simulink model "ZOP_Main"  (R2018b)
settings: Solver=FixedStepDiscrete  StartTime=0.0  StopTime=inf  FixedStep=0.01  RelTol=1e-3
PostLoadFcn:
  | if any(exist('dsrtsu_mdlpostloadfcn', 'file') ~= 0), dsrtsu_mdlpostloadfcn('Execute', bdroot); end
values from neighbouring files (symbols this model uses):
  k_ZOP_ALC_Ramp = 1.0    [ZOP_Func.sldd]
  k_ZOP_LS_ChangingDist = 5.0    [ZOP_Func.sldd]
  k_ZOP_LS_ChangingTime = 0.5    [ZOP_Func.sldd]
  k_ZOP_SpdLmt_Enable = 1.0    [ZOP_Func.sldd]
  k_ZOP_V2X_Enable = 1.0    [ZOP_Func.sldd]
  k_ZOP_VcTJA_Enable = 1.0    [ZOP_Func.sldd]
  k_ZOP_VoiceAct_Enable = 1.0    [ZOP_Func.sldd]
  MODE_ZOP_ACTIVE = 3.0    [ZOP_Func.sldd]
  MODE_ZOP_FINISH = 10.0    [ZOP_Func.sldd]
  MODE_ZOP_LC = 7.0    [ZOP_Func.sldd]
(part 2 of 2)

== stateflow chart ZOP_Main/ZOP_Main_OS/ZOP_State_Machine ==
  state OFF
    en:
    ZOP_Mode = MODE_ZOP_OFF;
  state PASSIVE
    en:
    ZOP_Mode = MODE_ZOP_PASSIVE;
    ZOP_Vars = InitHoldState(ZOP_Vars);
    du:
    ZOP_Ready = CheckZopPreCondition(SystemCmd, VehStatus, MapInfo,...
    ACC_Status, LKS_Status);
  state FINISH
    en:
    ZOP_Mode = MODE_ZOP_FINISH;
    finishTimeCnt = 0;
    du:
    finishTimeCnt++;
  state ERROR
    en:
    ZOP_Mode = MODE_ZOP_ERROR;
    du:
    ;
  state READY
    en:
    ZOP_Mode = MODE_ZOP_READY;
    LaneChangeCmd = 0; ZOP_Finish = 0;
    LCRefDir = 0; LCDesDir = 0;
    du:
    ZOP_Ready = CheckZopPreCondition(SystemCmd, VehStatus, MapInfo,...
    ACC_Status, LKS_Status);
  state ENABLE
    en:
    ;
    du:
    ;
    state HOLD
      en:
      ZOP_Mode = MODE_ZOP_HOLD;
      LaneChangeCmd = 0; ZOP_Finish = 0;
      ZOP_Vars = InitHoldState(ZOP_Vars);
      % CheckLCResult();
      du:
      ZOP_Ready = CheckZopPreCondition(SystemCmd, VehStatus, MapInfo,...
      ACC_Status, LKS_Status);
      [LaneChangeCmd, LaneChangeDir, ZOP_Finish, ZOP_Vars] = CheckZopLCCondition(VehStatus, FusionObj,...
      FusionLane, MapInfo, RoadModel_Lane, RoadModel_TS, TgtObj, FObj, ZOP_Vars);
    state OVERIDE
      en:
      ZOP_Mode = MODE_ZOP_OVERIDE;
      du:
      ;
    state LANE_CHANGE
      en:
      ZOP_Mode = MODE_ZOP_LC;
      LaneChangeQuit = 0;
      ZOP_Vars = InitLCState(ZOP_Vars);
      du:
      [LaneChangeQuit, ZOP_Vars] = CheckZopLC(LaneChangeCmd, FusionObj,...
      FusionLane, MapInfo, RoadModel_Lane, LKS_Status, TgtObj, ZOP_Vars);
    (default) -> HOLD
    HOLD -> LANE_CHANGE [order 2] : [LaneChangeCmd == -1 || ...
        | LaneChangeCmd == 1]
    HOLD -> OVERIDE [order 1] : [ACC_Status.overide == 1 || ...
        | LKS_Status.overide == 1]
    LANE_CHANGE -> HOLD : [LaneChangeQuit]
    OVERIDE -> HOLD : [ACC_Status.overide == 0 && ...
        | LKS_Status.overide == 0]
  (default) -> OFF
  ERROR -> OFF [order 2] : [SystemCmd.SystemOn != 1]
  ENABLE -> OFF [order 4] : [SystemCmd.SystemOn != 1]
  READY -> OFF [order 1] : [SystemCmd.SystemOn != 1]
  FINISH -> OFF [order 1] : [SystemCmd.SystemOn != 1]
  OFF -> PASSIVE : [SystemCmd.SystemOn == 1]
  PASSIVE -> OFF [order 1] : [SystemCmd.SystemOn != 1]
  FINISH -> PASSIVE [order 2] : [finishTimeCnt >= 50]
  PASSIVE -> READY [order 2] : [ZOP_Ready == 1]
  READY -> PASSIVE [order 2] : [ZOP_Ready != 1]
  ENABLE -> FINISH [order 3] : [ZOP_Finish]
  ERROR -> READY [order 1] : [ACC_Status.error == 0 && ...
      | LKS_Status.error == 0]
  READY -> ERROR [order 3] : [ACC_Status.error == 1 || ...
      | LKS_Status.error == 1]
  READY -> ENABLE [order 4] : [ZOP_Ready == 1 ...
      | && SystemCmd.SystemEnable == 1 ...
      | && SystemCmd.SystemCancel != 1]
  ENABLE -> READY [order 2] : [ZOP_Ready != 1 ...
      | || SystemCmd.SystemCancel == 1]
  ENABLE -> ERROR [order 1] : [ACC_Status.error == 1 || ...
      | LKS_Status.error == 1]
  data: SystemCmd function_input Bus: SystemCmd_ST; VehStatus function_input Bus: VSI_VEHSTATE_ST; MapInfo function_input Bus: MapInfo_ST_Post; zop_ready function_output double; ACC_Status function_input Bus: ACC_Status_ST; LKS_Status function_input Bus: LKS_Status_ST; ZOPVars_in function_input Bus: ZOP_Var_ST; ZOPVars function_output Bus: ZOP_Var_ST; ZOPVars_in function_input Bus: ZOP_Var_ST; ZOPVars function_output Bus: ZOP_Var_ST; VehStatus function_input Bus: VSI_VEHSTATE_ST; FusionObj function_input Bus: FUS_OBJ_OUTPUT_ST; FusionLane function_input Bus: FUS_LANE_OUTPUT_ST; MapInfo function_input Bus: MapInfo_ST_Post; lc_cmd function_output int8; lc_pro function_output int8; ZOP_Finish function_output int8; RoadModel_Lane function_input Bus: LANEMODEL_OUTPUT_ST; RoadModel_TS function_input Bus: HWA_TARGETOBJECT_OUTPUT_ST; TgtObj function_input Bus: ZOP_Object_ST size=8; FObj function_input Bus: ZOP_Object_ST; ZOPVars_in function_input Bus: ZOP_Var_ST; ZOPVars function_output Bus: ZOP_Var_ST; k_ZOP_ALC_Enable parameter; k_ZOP_HoldCnt parameter; k_ZOP_LCProCnt parameter; k_ZOP_ALC_D10 parameter; k_ZOP_MapFlag_Enable parameter; k_ZOP_ALC_SCnt parameter; k_ZOP_ALC_SNCnt parameter; k_ZOP_ALC_SCnt_Thr parameter; k_ZOP_ALC_SpdEnable parameter; k_ZOP_SpdCkDstThr parameter; k_ZOP_ObjSpd_cf parameter; k_ZOP_SpdLoThr parameter; k_ZOP_SpdLoTimeThr parameter; k_ZOP_ALC_Ramp parameter; LCCmd function_input int8; FusionObj function_input Bus: FUS_OBJ_OUTPUT_ST; FusionLane function_input Bus: FUS_LANE_OUTPUT_ST; MapInfo function_input Bus: MapInfo_ST_Post; LC_Quit function_output int8; RoadModel_Lane function_input Bus: LANEMODEL_OUTPUT_ST; LKS_Status function_input Bus: LKS_Status_ST; TgtObj function_input Bus: ZOP_Object_ST size=8; ZOPVars_in function_input Bus: ZOP_Var_ST; ZOPVars function_output Bus: ZOP_Var_ST; k_ZOP_LCTimeMax parameter; k_ZOP_ALC_SCnt_LC parameter; k_ZOP_ALC_SNCnt_LC parameter; k_ZOP_ALC_SCnt_Thr_LC parameter; SystemCmd input Bus: SystemCmd_ST; VehStatus input Bus: VSI_VEHSTATE_ST; FusionObj input Bus: FUS_OBJ_OUTPUT_ST; FusionLane input Bus: FUS_LANE_OUTPUT_ST; RoadModel_Lane input Bus: LANEMODEL_OUTPUT_ST; RoadModel_TS input Bus: HWA_TARGETOBJECT_OUTPUT_ST; MapInfo input Bus: MapInfo_ST_Post; ACC_Status input Bus: ACC_Status_ST; LKS_Status input Bus: LKS_Status_ST; ZOP_Ready local int8; holdTimeCnt local int8; finishTimeCnt local int8; LaneChangeQuit local int8; LC_Succ local int8; LC_Fail local int8; lcTimeCnt local int8; ZOP_Mode output int8; ZOP_Finish output int8; LCPlanningState local int8; LaneChangeDcsn local int8; MODE_ZOP_ERROR parameter double; MODE_ZOP_FINISH parameter double; MODE_ZOP_HOLD parameter; MODE_ZOP_LC parameter; MODE_ZOP_OFF parameter; MODE_ZOP_OVERIDE parameter; MODE_ZOP_PASSIVE parameter; LCRefDir local int8; LCDesDir local int8; ZOP_Vars output Bus: ZOP_Var_ST; MODE_ZOP_READY parameter; TgtObj input Bus: ZOP_Object_ST size=8; LaneChangeCmd output int8; LaneChangeDir output int8; FObj input Bus: ZOP_Object_ST
  function zop_ready  = CheckZopPreCondition(SystemCmd, VehStatus, MapInfo,...:
    | function zop_ready  = CheckZopPreCondition(SystemCmd, VehStatus, MapInfo,...
    |     ACC_Status, LKS_Status)
    | 
    | zop_ready = 0;
    | if MapInfo.isInZopZone == 1 && (ACC_Status.ready || ACC_Status.active)...
    |         && (LKS_Status.ready || LKS_Status.active) % gear = D
    |     zop_ready = 1;
    | end
  function ZOPVars = InitHoldState(ZOPVars_in):
    | function ZOPVars = InitHoldState(ZOPVars_in)
    | 
    | ZOPVars = ZOPVars_in;
    | ZOPVars.LCRes = uint16(0);
    | ZOPVars.LCTip = uint16(0);
    | ZOPVars.LCNRes = uint16(0);
    | ZOPVars.DesLane = int8(0);
    | ZOPVars.LCDir = int8(0);
    | ZOPVars.holdTimeCnt = uint32(0);
    | ZOPVars.lcTimeCnt = uint32(0);
    | ZOPVars.lcProTimeCnt = uint32(0);
    | ZOPVars.lcDirCnt = uint32(0);
    | ZOPVars.Safe = int8(0);
    | ZOPVars.LSafeRaw = int8(0);
    | ZOPVars.LSafeCnt = int8(0);
    | ZOPVars.LSafeNCnt = int8(0);
    | ZOPVars.RSafeRaw = int8(0);
    | ZOPVars.RSafeCnt = int8(0);
    | ZOPVars.RSafeNCnt = int8(0);
    | ZOPVars.FinishState = int8(0);
    | ZOPVars.LCFailTip = int8(0);
    | ZOPVars.SpdTimeCnt(:) = uint32(0);
    | ZOPVars.SpdTmp(:) = single(100/3.6);
    | ZOPVars.Spd(:) = single(0/3.6);
    | ZOPVars.MapFlagDir = int8(0);
    | %ZOPVars.MapFlag = uint16(0);
  function ZOPVars = InitLCState(ZOPVars_in):
    | function ZOPVars = InitLCState(ZOPVars_in)
    | 
    | ZOPVars = ZOPVars_in;
    | ZOPVars.lcTimeCnt = uint32(0);
    | ZOPVars.Safe = int8(0);
    | ZOPVars.LSafeRaw = int8(0);
    | ZOPVars.LSafeCnt = int8(0);
    | ZOPVars.LSafeNCnt = int8(0);
    | ZOPVars.RSafeRaw = int8(0);
    | ZOPVars.RSafeCnt = int8(0);
    | ZOPVars.RSafeNCnt = int8(0);
    | ZOPVars.LCFailTip = int8(0);
  function [lc_cmd, lc_pro, ZOP_Finish, ZOPVars] = CheckZopLCCondition(VehStatus, FusionObj,...:
    | function [lc_cmd, lc_pro, ZOP_Finish, ZOPVars] = CheckZopLCCondition(VehStatus, FusionObj,...
    |     FusionLane, MapInfo, RoadModel_Lane, RoadModel_TS, TgtObj, FObj, ZOPVars_in)
    | 
    | ZOPVars = ZOPVars_in;
    | ZOPVars.LCRes = uint16(0);
    | ZOPVars.LCNRes = uint16(0);
    | ZOPVars.DesLane = int8(0);
    | ZOPVars.LCDir = int8(0);
    | ZOPVars.LCTime = single(8);
    | ZOPVars.LCCmd = int8(0);
    | lc_cmd = int8(0);
    | lc_pro = int8(0);
    | ZOP_Finish = int8(0);
    | ZOPVars.MapFlagDir = int8(0);
    | 
    | ZOPVars.LnHi = MapInfo.LaneNum;
    | ZOPVars.LnLo = int8(1);
    | if MapInfo.Dist2Dest > 3000
    |     ZOPVars.LnLo = min(MapInfo.LaneNum,min(2,MapInfo.LaneNum/2+1));
    |     %ZOPVars.DesLane = max(min(2,MapInfo.LaneNum), MapInfo.LaneIndex);
    | 	if MapInfo.Dist2Dest > 4000
    |         %ZOPVars.DesLane = max(int8(MapInfo.LaneNum/2+1),MapInfo.LaneIndex);
    |         ZOPVars.LnLo = min(MapInfo.LaneNum,int8(MapInfo.LaneNum/2+1));
    |     end
    | elseif MapInfo.Dist2Dest > 2500
    |     ZOPVars.LnHi = min(MapInfo.LaneNum,int8(MapInfo.LaneNum/2+1));
    |     %ZOPVars.DesLane = min(int8(MapInfo.LaneNum/2+1),MapInfo.LaneIndex);
    | else
    |     ZOPVars.LnHi = min(2,MapInfo.LaneNum);
    |     %ZOPVars.DesLane = min(2, MapInfo.LaneIndex);
    | 	if MapInfo.Dist2Dest < k_ZOP_ALC_D10
    |         ZOPVars.LnHi = int8(1);
    |         %ZOPVars.DesLane = int8(1);
    |     end
    | end
    | if MapInfo.Dist2Dest < 65534
    |     if MapInfo.LaneIndex < ZOPVars.LnLo
    |         ZOPVars.LCDir = int8(-1);
    |         ZOPVars.LCRes = uint16(4);
    |         ZOPVars.LCTip = uint16(5);
    |     elseif MapInfo.LaneIndex > ZOPVars.LnHi
    |         ZOPVars.LCDir = int8(1);
    |         ZOPVars.LCRes = uint16(2);
    |         ZOPVars.LCTip = uint16(3);
    |     end
    | end
    | 
    | % TODO:spd
    | ZOPVars.SpdTmp(:) = single(100/3.6);
    | if FObj.id > 0.5 && FObj.x < k_ZOP_SpdCkDstThr
    |     ZOPVars.SpdTmp(1) = FObj.vx+VehStatus.vRef;
    | end
    | for i=1:8
    |     if TgtObj(i).dir_f > 0 && TgtObj(i).dir < 0 && TgtObj(i).x < k_ZOP_SpdCkDstThr
    |         ZOPVars.SpdTmp(2) = min(ZOPVars.SpdTmp(2), TgtObj(i).vx+VehStatus.vRef);
    |     end
    |     if TgtObj(i).dir_f > 0 && TgtObj(i).dir > 0 && TgtObj(i).x < k_ZOP_SpdCkDstThr
    |         ZOPVars.SpdTmp(3) = min(ZOPVars.SpdTmp(3), TgtObj(i).vx+VehStatus.vRef);
    |     end
    | end
    | ZOPVars.Spd(1) = ZOPVars.SpdTmp(1)*k_ZOP_ObjSpd_cf + ZOPVars.Spd(1)*(1-k_ZOP_ObjSpd_cf);
    | ZOPVars.Spd(2) = ZOPVars.SpdTmp(2)*k_ZOP_ObjSpd_cf + ZOPVars.Spd(2)*(1-k_ZOP_ObjSpd_cf);
    | ZOPVars.Spd(3) = ZOPVars.SpdTmp(3)*k_ZOP_ObjSpd_cf + ZOPVars.Spd(3)*(1-k_ZOP_ObjSpd_cf);
    | if k_ZOP_ALC_SpdEnable > 0.5 && ZOPVars.LCDir == 0
    |     if ZOPVars.Spd(1) + k_ZOP_SpdLoThr < ZOPVars.Spd(2)
    |         ZOPVars.SpdTimeCnt(1) = ZOPVars.SpdTimeCnt(1) + uint32(1);
    |     else
    |         ZOPVars.SpdTimeCnt(1) = uint32(0);
    |     end
    |     if ZOPVars.Spd(1) + k_ZOP_SpdLoThr < ZOPVars.Spd(3)
    |         ZOPVars.SpdTimeCnt(2) = ZOPVars.SpdTimeCnt(2) + uint32(1);
    |     else
    |         ZOPVars.SpdTimeCnt(2) = uint32(0);
    |     end
    |     if ZOPVars.SpdTimeCnt(1) > k_ZOP_SpdLoTimeThr && MapInfo.LaneIndex+1 <= ZOPVars.LnHi
    |         ZOPVars.LCDir = int8(-1);
    |         ZOPVars.LCRes = uint16(1);
    |         ZOPVars.LCTip = uint16(1);
    |     % elseif ZOPVars.SpdTimeCnt(1) > k_ZOP_SpdLoTimeThr && MapInfo.LaneIndex+1 <= ZOPVars.LnHi
    |     end
    | end
    | 
    | % Ramp
    | if k_ZOP_ALC_Ramp > 0.5
    | %    if MapInfo.MapFlag ~= ZOPVars.MapFlag && (MapInfo.MapFlag == 1 || MapInfo.MapFlag == 2)
    |         if MapInfo.MapFlag == 1
    |             ZOPVars.MapFlagDir = int8(-1);
    |         elseif MapInfo.MapFlag == 2
    |             ZOPVars.MapFlagDir = int8(1);
    |         end
    | %    end
    |     if ZOPVars.MapFlagDir == -1 || ZOPVars.MapFlagDir == 1
    |         ZOPVars.LCDir = ZOPVars.MapFlagDir;
    | %         ZOPVars.LCCmd = ZOPVars.MapFlagDir;
    | %         lc_pro = ZOPVars.MapFlagDir;        
    |         ZOPVars.LCRes = uint16(2);
    |         ZOPVars.LCTip = uint16(3);
    | %         ZOPVars.lcProTimeCnt = ZOPVars.lcProTimeCnt + 1;
    | %         if ZOPVars.lcProTimeCnt > k_ZOP_LCProCnt/2
    | %             lc_cmd = ZOPVars.LCCmd;
    | %         end
    |     end
    |     ZOPVars.MapFlag = MapInfo.MapFlag;
    | else
    |     ZOPVars.MapFlag = uint16(0);
    | end
    | 
    | if k_ZOP_ALC_Ramp < 0.5 || ZOPVars.MapFlagDir == 0
    |     if MapInfo.LaneStable ~= 1
    |         ZOPVars.LCDir = int8(0);
    |         ZOPVars.LCNRes = ZOPVars.LCNRes + 1;
    |     end
    | end
    | if ZOPVars.LCDir == -1 && FusionLane.leftHostLane.type ~= 2 && ...
    |         FusionLane.leftHostLane.type ~= 6 && FusionLane.leftHostLane.type ~= 7
    |     ZOPVars.LCDir = int8(0);
    |     ZOPVars.LCNRes = ZOPVars.LCNRes + 2;
    | elseif ZOPVars.LCDir == 1 && FusionLane.rightHostLane.type ~= 2 && ...
    |         FusionLane.rightHostLane.type ~= 5 && FusionLane.rightHostLane.type ~= 7
    |     ZOPVars.LCDir = int8(0);
    |     ZOPVars.LCNRes = ZOPVars.LCNRes + 2;
    | end
    | 
    | ZOPVars.Safe = int8(0);
    | ZOPVars.LSafeRaw = int8(1);
    | ZOPVars.RSafeRaw = int8(1);
    | for i=1:8
    |     if TgtObj(i).dir == -1 && (TgtObj(i).exist(1) == 1 || TgtObj(i).exist(2) == 1)
    |         ZOPVars.LSafeRaw = int8(0);
    |     elseif TgtObj(i).dir == 1 && (TgtObj(i).exist(1) == 1 || TgtObj(i).exist(2) == 1)
    |         ZOPVars.RSafeRaw = int8(0);
    |     end
    | end
    | if ZOPVars.LSafeRaw == 1
    |     ZOPVars.LSafeCnt = min(ZOPVars.LSafeCnt+1, k_ZOP_ALC_SCnt);
    |     ZOPVars.LSafeNCnt = max(ZOPVars.LSafeNCnt-1, 0);
    | else
    |     ZOPVars.LSafeCnt = max(ZOPVars.LSafeCnt-1, 0);
    |     ZOPVars.LSafeNCnt = min(ZOPVars.LSafeNCnt+1, k_ZOP_ALC_SNCnt);
    | end
    | if ZOPVars.RSafeRaw == 1
    |     ZOPVars.RSafeCnt = min(ZOPVars.RSafeCnt+1, k_ZOP_ALC_SCnt);
    |     ZOPVars.RSafeNCnt = max(ZOPVars.RSafeNCnt-1, 0);
    | else
    |     ZOPVars.RSafeCnt = max(ZOPVars.RSafeCnt-1, 0);
    |     ZOPVars.RSafeNCnt = min(ZOPVars.RSafeNCnt+1, k_ZOP_ALC_SNCnt);
    | end
    | 
    | % if ZOPVars.SafeCnt > 20 && ZOPVars.SafeNCnt <= 5
    | %     ZOPVars.Safe = int8(1);
    | % elseif ZOPVars.SafeNCnt > 20 && ZOPVars.SafeCnt <= 5
    | %     ZOPVars.Safe = int8(-1);
    | % end
    | 
    | if ZOPVars.LCDir == -1
    |     if ZOPVars.LSafeCnt > k_ZOP_ALC_SCnt_Thr && ZOPVars.LSafeNCnt <= 3 && ZOPVars.LSafeRaw == 1
    |         %ZOPVars.Safe = int8(0);        
    |     else
    |         %ZOPVars.Safe = int8(-1);
    |         ZOPVars.LCDir = int8(0);
    |         ZOPVars.LCNRes = ZOPVars.LCNRes + 4;
    |     end
    | elseif ZOPVars.LCDir == 1
    |     if ZOPVars.RSafeCnt > k_ZOP_ALC_SCnt_Thr && ZOPVars.RSafeNCnt <= 3 && ZOPVars.RSafeRaw == 1
    |         %ZOPVars.Safe = int8(0);        
    |     else
    |         %ZOPVars.Safe = int8(-1);
    |         ZOPVars.LCDir = int8(0);
    |         ZOPVars.LCNRes = ZOPVars.LCNRes + 4;
    |     end
    | end
    | 
    | % if ZOPVars.Safe == 0
    | %     ZOPVars.LCDir = int8(0);
    | %     ZOPVars.LCNRes = ZOPVars.LCNRes + 4;
    | % end
    | % if ZOPVars.Safe == -1
    | %     ZOPVars.LCDir = int8(0);
    | %     ZOPVars.LCNRes = ZOPVars.LCNRes + 4;
    | % end
    | 
    | % time check
    | ZOP_HoldCnt = k_ZOP_HoldCnt;
    | if k_ZOP_ALC_Ramp > 0.5
    |     if MapInfo.MapFlag ~= 0
    |         ZOP_HoldCnt = single(10);
    |     else
    |         ZOP_HoldCnt = single(30);
    |     end
    | end
    | if ZOPVars.LCDir == 1 || ZOPVars.LCDir == -1
    |     if ZOPVars.holdTimeCnt > ZOP_HoldCnt
    |         ZOPVars.LCCmd = ZOPVars.LCDir;
    |         ZOPVars.lcDirCnt = ZOPVars.lcDirCnt+1;
    |     else
    |         ZOPVars.LCCmd = int8(0);
    |         ZOPVars.LCNRes = ZOPVars.LCNRes + 8;
    |     end
    | end
    | if MapInfo.MapFlag ~= 0 && k_ZOP_MapFlag_Enable > 0.5
    |     ZOPVars.LCCmd = int8(0);
    |     ZOPVars.LCNRes = ZOPVars.LCNRes + 256;
    | end
    | 
    | if ZOPVars.LCCmd == -1 || ZOPVars.LCCmd == 1
    |     lc_pro = ZOPVars.LCCmd;
    |     ZOPVars.lcProTimeCnt = ZOPVars.lcProTimeCnt + 1;
    | else
    |     ZOPVars.lcProTimeCnt = uint32(0);    
    |     ZOPVars.LCRes = uint16(0);
    |     ZOPVars.LCTip = uint16(0);
    | end
    | if (ZOPVars.lcProTimeCnt > k_ZOP_LCProCnt) || (k_ZOP_ALC_Ramp > 0.5 &&...
    |         ZOPVars.MapFlagDir ~= 0 && ZOPVars.lcProTimeCnt > k_ZOP_LCProCnt/3)
    |     lc_cmd = ZOPVars.LCCmd;
    | end
    | if k_ZOP_ALC_Enable < 0.5
    |     lc_cmd = int8(0);
    |     lc_pro = int8(0);
    |     ZOPVars.LCRes = uint16(0);
    |     ZOPVars.LCTip = uint16(0);
    | end
    | 
    | if k_ZOP_ALC_Ramp > 0.5
    |     if MapInfo.MapFlag == 128
    |         ZOPVars.FinishState = int8(1);
    |     end
    | else
    |     % Fail
    |     if (MapInfo.LocIndex == 1 || MapInfo.LocIndex == 3) && MapInfo.Dist2Dest < 400  && MapInfo.LaneIndex > 1
    |         ZOPVars.FinishState = int8(2);    % takeover
    |     elseif (MapInfo.LocIndex == 1 || MapInfo.LocIndex == 3) && MapInfo.Dist2Dest < 300  && MapInfo.LaneIndex == 1
    |         ZOPVars.FinishState = int8(1);
    |     end
    | end
    | ZOP_Finish = ZOPVars.FinishState;
    | ZOPVars.holdTimeCnt = ZOPVars.holdTimeCnt+1;
  function [LC_Quit, ZOPVars] = CheckZopLC(LCCmd, FusionObj,...:
    | function [LC_Quit, ZOPVars] = CheckZopLC(LCCmd, FusionObj,...
    |     FusionLane, MapInfo, RoadModel_Lane, LKS_Status, TgtObj, ZOPVars_in)
    | 
    | ZOPVars = ZOPVars_in;
    | ZOPVars.LCResult = int8(0);
    | 
    | ZOPVars.LSafeRaw = int8(1);
    | ZOPVars.RSafeRaw = int8(1);
    | for i=1:8
    |     if TgtObj(i).dir == -1 && (TgtObj(i).exist(1) == 1 || TgtObj(i).exist(2) == 1)
    |         ZOPVars.LSafeRaw = int8(0);
    |     elseif TgtObj(i).dir == 1 && (TgtObj(i).exist(1) == 1 || TgtObj(i).exist(2) == 1)
    |         ZOPVars.RSafeRaw = int8(0);
    |     end
    | end
    | if ZOPVars.LSafeRaw == 1
    |     ZOPVars.LSafeCnt = min(ZOPVars.LSafeCnt+1, k_ZOP_ALC_SCnt_LC);
    |     ZOPVars.LSafeNCnt = max(ZOPVars.LSafeNCnt-1, 0);
    | else
    |     ZOPVars.LSafeCnt = max(ZOPVars.LSafeCnt-1, 0);
    |     ZOPVars.LSafeNCnt = min(ZOPVars.LSafeNCnt+1, k_ZOP_ALC_SNCnt_LC);
    | end
    | if ZOPVars.RSafeRaw == 1
    |     ZOPVars.RSafeCnt = min(ZOPVars.RSafeCnt+1, k_ZOP_ALC_SCnt_LC);
    |     ZOPVars.RSafeNCnt = max(ZOPVars.RSafeNCnt-1, 0);
    | else
    |     ZOPVars.RSafeCnt = max(ZOPVars.RSafeCnt-1, 0);
    |     ZOPVars.RSafeNCnt = min(ZOPVars.RSafeNCnt+1, k_ZOP_ALC_SNCnt_LC);
    | end
    | 
    | if LKS_Status.lc_fail
    |     ZOPVars.LCResult = int8(-1);
    |     ZOPVars.LCFailTip = int8(4);
    | elseif LKS_Status.lc_finish
    |     ZOPVars.LCResult = int8(1);
    | elseif ZOPVars.lcTimeCnt*0.1 > k_ZOP_LCTimeMax
    |     ZOPVars.LCResult = int8(-1);
    | else
    |     if LCCmd == -1
    |         if ZOPVars.LSafeNCnt >= k_ZOP_ALC_SCnt_Thr_LC && ZOPVars.LSafeCnt <= 5 && ZOPVars.LSafeRaw == 0
    |             ZOPVars.LCResult = int8(-1);
    |             ZOPVars.LCFailTip = int8(1);
    |         end
    | %         for i=1:8
    | %             if TgtObj(i).dir == -1 && TgtObj(i).exist(2) == 1
    | %                 ZOPVars.LCResult = int8(-1);
    | %                 break;
    | %             end
    | %         end
    |     elseif LCCmd == 1
    |         if ZOPVars.RSafeNCnt >= k_ZOP_ALC_SCnt_Thr_LC && ZOPVars.RSafeCnt <= 5 && ZOPVars.RSafeRaw == 0
    |             ZOPVars.LCResult = int8(-1);
    |             ZOPVars.LCFailTip = int8(1);
    |         end
    | %         for i=1:8
    | %             if TgtObj(i).dir == 1 && TgtObj(i).exist(2) == 1
    | %                 ZOPVars.LCResult = int8(-1);
    | %                 break;
    | %             end
    | %         end
    |     end
    | end
    | 
    | ZOPVars.lcTimeCnt = ZOPVars.lcTimeCnt+1;
    | ZOPVars.LCDist = LKS_Status.lc_dist;
    | if ZOPVars.LCDist > 0 && ZOPVars.LCDist < 3.5
    |     ZOPVars.LCTime = 8*ZOPVars.LCDist/3.5;
    | else
    |     ZOPVars.LCTime = single(8);
    | end
    | 
    | if ZOPVars.LCResult ~= 0
    |     if ZOPVars.LCResult < 0
    |         ZOPVars.LCTip = uint16(7);
    |     end
    |     LC_Quit = int8(1);
    | else
    |     LC_Quit = int8(0);
    | end

== stateflow chart ZOP_Main/ZOP_OS ==
  settings: sampleTime=0.005
  (default) -> (junction 1) : {
      | i = i+1;
      | }
  (junction 1) -> (junction 22) [order 1] : [i %% 2 == 0]
  (junction 22) -> (junction 4) : {
      | do_ZOP_CAN;
      | do_LightLogic;
      | }
  (junction 1) -> (junction 4) [order 2]
  (junction 4) -> (junction 7) [order 1] : [i >= 10]
  (junction 4) -> (junction 6) [order 2]
  (junction 7) -> (junction 8) : {
      | do_LKS_CONV;
      | do_ZOP_Feature;
      | i = 0;
      | }
  (junction 8) -> (junction 6)
  (junction 6) -> (junction 13)
  data: i local int32
  events: do_ZOP_CAN output FUNCTION_CALL_EVENT; do_LightLogic output FUNCTION_CALL_EVENT; do_ZOP_Feature output FUNCTION_CALL_EVENT; do_LKS_CONV output FUNCTION_CALL_EVENT

== stateflow chart ZOP_Main/ZOP_Main_OS/LaneStateProcess ==
  settings: description=_0p0.DUMMY.222_000_
  state STABLE
    en:
    LaneStable = (LaneCur != 0);
    LaneCurPost = LaneCur;
    du:
    LaneStable = (LaneCur != 0);
  state CHANGING
    en:
    LaneStable = 0;
    changingCnt = 0;
    du:
    changingCnt++;
  state INIT
    en:
    LaneStable = 0;
    LaneCurPost = LaneCur;
  STABLE -> INIT [order 1] : [!ZOP_Enable]
  STABLE -> CHANGING [order 2] : [LaneNum_last != LaneNum ...
      | || LaneCur_last != LaneCur ...
      | || LCState == MODE_ZOP_LC]
  CHANGING -> STABLE [order 2] : [changingCnt*0.1 > k_LS_ChangingTime ...
      | && VehSpeed_mps*changingCnt*0.1 > k_LS_ChangingDist]
  CHANGING -> CHANGING [order 1] : [LaneCur_last != LaneCur ...
      | || LaneNum_last != LaneNum ...
      | || LCState == MODE_ZOP_LC]
  INIT -> CHANGING : [ZOP_Enable]
  CHANGING -> INIT [order 3] : [!ZOP_Enable]
  (default) -> INIT
  data: ZOP_Enable input; LaneCurPost output; changingCnt local int32; LaneCur input; LaneCur_last input; LCState input; VehSpeed_mps input; LaneStable output; LaneNum input; LaneNum_last input; k_LS_ChangingDist input; k_LS_ChangingTime input; MODE_ZOP_LC parameter

== stateflow chart ZOP_Main/ZOP_Main_OS/TargetCheck ==
  state DEFAULT
    en:
    ;
    du:
    [ObjTarget, ObjNum] = GetTarget(VehStatus, FusionObj, ...
    FusionLane, RoadModel_Lane, RoadModel_TS, LC_Time, ObjTarget);
    state [TargetExist,TargetExist2] = CheckTargetR(LC_Time,VehStatus,Object) [function]
    state [TargetExist,TargetExist2] = CheckTargetF(LC_Time,VehStatus,Object) [function]
  (default) -> DEFAULT
  data: VehStatus function_input Bus: VSI_VEHSTATE_ST; FusionObj function_input Bus: FUS_OBJ_OUTPUT_ST; FusionLane function_input Bus: FUS_LANE_OUTPUT_ST; Objects function_output Bus: ZOP_Object_ST size=8; RoadModel_Lane function_input Bus: LANEMODEL_OUTPUT_ST; RoadModel_TS function_input Bus: HWA_TARGETOBJECT_OUTPUT_ST; LC_Time function_input double; ObjNum function_output int8; Objects_in function_input Bus: ZOP_Object_ST size=8; LC_Time function_input double; VehStatus function_input Bus: VSI_VEHSTATE_ST; Object function_input Bus: ZOP_Object_ST; TargetExist function_output; TargetExist2 function_output; LC_Time function_input double; VehStatus function_input Bus: VSI_VEHSTATE_ST; Object function_input Bus: ZOP_Object_ST; TargetExist function_output; TargetExist2 function_output; VehStatus input Bus: VSI_VEHSTATE_ST; FusionObj input Bus: FUS_OBJ_OUTPUT_ST; FusionLane input Bus: FUS_LANE_OUTPUT_ST; RoadModel_Lane input Bus: LANEMODEL_OUTPUT_ST; RoadModel_TS input Bus: HWA_TARGETOBJECT_OUTPUT_ST; ObjTarget output Bus: ZOP_Object_ST size=8; LC_Time input; ObjNum output double
  function [Objects, ObjNum] = GetTarget(VehStatus, FusionObj,...:
    | function [Objects, ObjNum] = GetTarget(VehStatus, FusionObj,...
    |     FusionLane, RoadModel_Lane, RoadModel_TS, LC_Time, Objects_in)
    | 
    | OBJ_NUM_MAX = 40;
    | ObjNum=int8(0);
    | Objects = Objects_in;
    | ids = zeros(8,1);
    | indexs = zeros(8,1);
    | ids(1) = RoadModel_TS.L_NEIGHBORLANE_TAROBJ_0_ST.ID_un8;
    | ids(2) = RoadModel_TS.L_NEIGHBORLANE_TAROBJ_1_ST.ID_un8;
    | ids(3) = RoadModel_TS.L_NEIGHBORLANE_TAROBJ_2_ST.ID_un8;
    | ids(4) = RoadModel_TS.L_NEIGHBORLANE_TAROBJ_3_ST.ID_un8;
    | ids(5) = RoadModel_TS.R_NEIGHBORLANE_TAROBJ_0_ST.ID_un8;
    | ids(6) = RoadModel_TS.R_NEIGHBORLANE_TAROBJ_1_ST.ID_un8;
    | ids(7) = RoadModel_TS.R_NEIGHBORLANE_TAROBJ_2_ST.ID_un8;
    | ids(8) = RoadModel_TS.R_NEIGHBORLANE_TAROBJ_3_ST.ID_un8;
    | indexs(1) = RoadModel_TS.L_NEIGHBORLANE_TAROBJ_0_ST.Index_un8;
    | indexs(2) = RoadModel_TS.L_NEIGHBORLANE_TAROBJ_1_ST.Index_un8;
    | indexs(3) = RoadModel_TS.L_NEIGHBORLANE_TAROBJ_2_ST.Index_un8;
    | indexs(4) = RoadModel_TS.L_NEIGHBORLANE_TAROBJ_3_ST.Index_un8;
    | indexs(5) = RoadModel_TS.R_NEIGHBORLANE_TAROBJ_0_ST.Index_un8;
    | indexs(6) = RoadModel_TS.R_NEIGHBORLANE_TAROBJ_1_ST.Index_un8;
    | indexs(7) = RoadModel_TS.R_NEIGHBORLANE_TAROBJ_2_ST.Index_un8;
    | indexs(8) = RoadModel_TS.R_NEIGHBORLANE_TAROBJ_3_ST.Index_un8;
    | 
    | 
    | for i=1:8
    | %     if ids(i)==0
    | %         continue;
    | %     end
    |     Objects(i).id = uint8(0);
    |     Objects(i).exist = int8(zeros(2,1));
    |     Objects(i).x = single(0);
    |     Objects(i).y = single(0);
    |     Objects(i).vx = single(0);
    |     Objects(i).vy = single(0);
    |     Objects(i).ax = single(0);
    |     Objects(i).ay = single(0);
    |     Objects(i).dir = int8(0);
    |     Objects(i).dir_f = int8(0);
    |     for j=1:OBJ_NUM_MAX
    |         if FusionObj.objects(j).obj_property.id == ids(i)
    |             if FusionObj.objects(j).obj_information.valid ~= 1
    |                 break;
    |             end
    |             Objects(i).id = FusionObj.objects(j).obj_property.id;
    |             Objects(i).x = FusionObj.objects(j).obj_estimate.longPosition;
    |             Objects(i).y = FusionObj.objects(j).obj_estimate.latPosition;
    |             Objects(i).vx = FusionObj.objects(j).obj_estimate.longRelativeVelocity;
    |             Objects(i).vy = FusionObj.objects(j).obj_estimate.latRelativeVelocity;
    |             Objects(i).ax = FusionObj.objects(j).obj_estimate.longRelativeAcceleration;
    |             Objects(i).ay = FusionObj.objects(j).obj_estimate.latRelativeAcceleration;
    |             if Objects(i).y < 0 
    |                 Objects(i).dir = int8(1);
    |             else
    |                 Objects(i).dir = int8(-1);
    |             end
    |             if Objects(i).x >= 0
    |                 Objects(i).dir_f = int8(1);
    |                 [Objects(i).exist(1), Objects(i).exist(2)] = CheckTargetF(LC_Time,VehStatus,Objects(i));
    |             else
    |                 Objects(i).dir_f = int8(-1);
    |                 [Objects(i).exist(1), Objects(i).exist(2)] = CheckTargetR(LC_Time,VehStatus,Objects(i));
    |             end
    |             ObjNum = ObjNum+int8(1);
    |         end
    |     end
    | end

== matlab function ZOP_Main/LKS_Mode_Conv/LKS_Input_Proc ==
  data: LKS_Output output Bus: LKS_Status_ST; mode_raw input; mode_raw_last input; LC_dx input
function LKS_Output = fcn(mode_raw, mode_raw_last, LC_dx)

LKS_Output.state = uint8(mode_raw);
LKS_Output.ready = uint8(0);
LKS_Output.active = uint8(0);
LKS_Output.overide = uint8(0);
LKS_Output.cancle = uint8(0);
LKS_Output.error = uint8(0);
LKS_Output.lc_finish = uint8(0);
LKS_Output.lc_fail = uint8(0);
switch LKS_Output.state
    case 0
        LKS_Output.error = uint8(1);
    case 3
        LKS_Output.ready = uint8(1);
    case 4
        LKS_Output.active = uint8(1);
    case 5
        LKS_Output.active = uint8(1);
    case 6
        LKS_Output.active = uint8(1);
end

if (mode_raw_last == 4 || mode_raw_last == 5 || mode_raw_last == 6) && ...
        (mode_raw ~= 4 && mode_raw ~= 5 && mode_raw ~= 6)
    LKS_Output.cancle = uint8(1);
end

if mode_raw_last == 5 || mode_raw_last == 6
    if mode_raw == 4
        LKS_Output.lc_finish = uint8(1);
    elseif mode_raw ~= 5 && mode_raw ~= 6
        LKS_Output.lc_fail = uint8(1);
    end
end

LKS_Output.lc_dist = single(abs(LC_dx));

== matlab function ZOP_Main/Light_Process/LightLogic ==
  data: v_des output; a_des output; traf_sign input; velocity input; dist input; time_in input; CONST_LIMIT input; dist output; case_num output; Flag input
function [v_des,a_des,dist,case_num] = intesec_cross( traf_sign, velocity, dist, time_in,CONST_LIMIT,Flag)  
%% this is a function that provide desired velocity, and distance to traffic light;
    % input: trafic_sign with green = 0; red = 1; yellow = 2;
    %        velocity in unit of kph;
    %        dist, and time is distance(m) to cross, and traffic time left
    %        CONST_LIMIT is velocity limit at cross, which is a reference CONSTANT velocity from
    %        ACC module.
    %        v_des_pre preseve previous v_des for next step use.
    
    % output: desired velocity for ACC module, in unit of kph;
    %         dist is distance(m) to front cross;
   
    case_num = 0;
    time = time_in;
    green = 1;
    red = 3;
    yellow = 2;
%     if time == 2
%         a_des = 0;
%          v_des = 0;
%     end
    
    if (Flag == 0)
        v_des = velocity;
        a_des = 0.5;
        dist = dist;
        case_num = 0;
       
        
    else   %(Flag == 1)

        if dist < 0
            dist = 0; 
        end

        v = velocity;

        if traf_sign == green
            time = time + 3;
        elseif traf_sign == yellow
            traf_sign = green;
        end

        switch traf_sign
            case green
                T_ACC = (max(0,dist)+0.1) / (v + 0.0001);
                T_ACC_QUIT = (dist - 5) / (v + 0.0001);
                T = time;
                a = 2 * (dist - v * T) / (T^2 + 0.0001);
                v_temp = v + a * T;
                
                if dist == 200
                    v_des = 15;
                    a_des = 1;
                    case_num = 0;
                    return;
                end
                
                if T_ACC_QUIT > 8  && v < 2.5
                    v_des = 15;
                    a_des = 1;
                    case_num = 0;
                    return;
                end

                if T_ACC < T % green time is long enough
                    if v > CONST_LIMIT %
                        a0 =  (CONST_LIMIT^2 - v^2) / (2*dist + 0.001);
                        a0 = max(a0,-1);
                        vt = sqrt(max(0,v^2 + 2 * a0 * dist));
                        t0 = (vt - v) / (a0);
                        
                        if t0 <= T % decelerate to vt is OK
                            v_des = vt; % (v + t0 * a0);
                            a_des = a0;
                            case_num = 1;
                        else 
                            v_des = v + T * a0;
                            a_des = a0;
                            case_num = 2;
                        end
                    else % green 
                        v_des = CONST_LIMIT;
                        a_des = (CONST_LIMIT - v)/T;
                        case_num = 3;
                    end
                    
                else % ( T_ACC >= T)
                    if ((a >= 0) && (a < 1) && (v_temp <= CONST_LIMIT))
                        v_des = CONST_LIMIT;
                        a_des = a;
                        case_num = 4;
                    else
                        v_des  = 0;
                        a_des = -v^2 / (2 * dist); 
                        case_num = 5;
                    end
                end

            case red
                T_ACC_QUIT = (dist - 5) / (v + 0.0001);
                if T_ACC_QUIT > 10 && dist >= 5
                    v_des = 15;
                    a_des = 1;
                    case_num = 0;
                    return;
                end

                if (dist < 4) && (v < 1)
                    a_des = 0.25 * dist - 1;
                    v_des = 0;
                    case_num = 12;

                else
                    T = time;
                    T_ACC = dist / (v + 0.0001);
                    a = 2 * (dist - v * T) / (T+0.001)^2;
                    v_temp = v + a * T;

                    if T_ACC < T
                        a0 = -v^2 / (2 * dist);
                        t0 = -v / a0;
                        if t0 < time
                            v_des = 0;
                            a_des = max(-1, -v^2 / (2 * dist+ 0.01));
                            case_num = 7;
                        else
                            v_des = v_temp;
                            a_des = a;
                            case_num = 8;
                        end 

                    else % (T_ACC > T)
                        if (v_temp < CONST_LIMIT)
                            v_des = v_temp;
                            a_des = max(-1,a);
                            case_num = 9;
                        else
                            v_des = CONST_LIMIT;
                            a_des = (CONST_LIMIT - v) / T;
                            case_num = 10;
                        end

                    end
                end

               

            otherwise
                v_des = CONST_LIMIT;
                a_des = 0;
                case_num = 11;
        end
        
%     else
%         v_des = 100;
%         a_des = 100;
%         dist = 100;
%         case_num = 0;
%          
    end
end
